simulink model "Tx_Rx"  (R2020a)
settings: Solver=VariableStepAuto  StartTime=0.0  StopTime=640e-9  RelTol=1e-3
libraries: msbUtilities x102, simulink_extras x15, dspswit3 x4, dspsigops x2
(part 1 of 3)
settings Model: Creator=lenovo  LastModifiedBy=dell

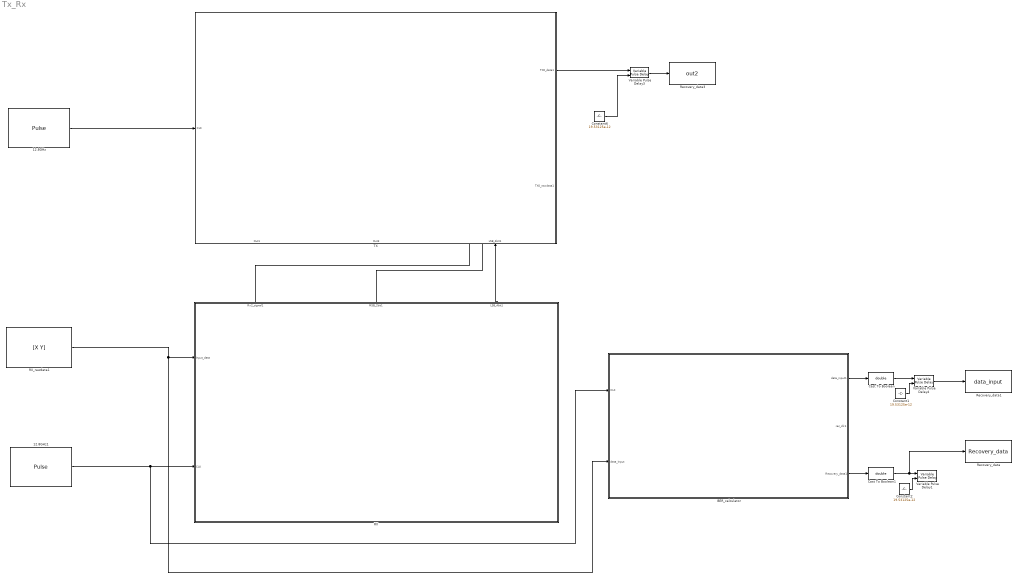
== system Tx_Rx ==
  12.8GHz : DiscretePulseGenerator  PulseType=Time based  Period=78.125e-12  PulseWidth=50
  12.8GHz1 : DiscretePulseGenerator  PulseType=Time based  Period=78.125e-12  PulseWidth=50
  BER_calculator : Subsystem
  Cast To Boolean : DataTypeConversion  OutDataTypeStr=double
  Cast To Boolean1 : DataTypeConversion  OutDataTypeStr=double
  Constant1 : Constant  Value=19.53125e-12
  Constant2 : Constant  Value=19.53125e-12
  Constant6 : Constant  Value=19.53125e-12
  RX : Subsystem
      settings: PortSchema="{\"entries\":[{\"content\":{\"sides\":[{\"content\":{\"connectorIds\":[]},\"type\":\"ConnectorPlacement.EquallySpacedRectSide\",\"uuid\":\"83fb874e-4081-4857-a545-3ede401996a7\"},{\"content\":{\"connectorIds\":[\"Out1\",\"Out2\",\"Out3\"],\"side\":\"RIGHT\"},\"type\":\"ConnectorPlacement.EquallySpacedRectSide\",\"uuid\":\"baf7f71f-d39c-46fb-b6e7-a302eb8d75df\"},{\"content\":{\"connectorIds\":[\"In1\",\"In2\"],\"side\":\"TOP\"},\"type\":\"ConnectorPlacement.EquallySpacedRectSide\",\"uuid\":\"afee1bbb-74d0-41b9-9455-dab1a6c8e3ec\"}]},\"type\":\"ConnectorPlacement.EquallySpacedConnector\",\"uuid\":\"642b16a5-7b6d-4c37-b7c9-a415dc76cc31\"}],\"packageUris\":[\"http://schema.mathworks.com/mf0/Connector/19700101\"],\"version\":\"1.0\"}"
  RX_rawdata1 : FromWorkspace  VariableName=[X Y]  SampleTime=1.220703125e-12  OutputAfterFinalValue=Setting to zero
  Recovery_data : ToWorkspace  VariableName=Recovery_data  SampleTime=39.0625e-12
  Recovery_data1 : ToWorkspace  VariableName=data_input  SampleTime=39.0625e-12
  Recovery_data3 : ToWorkspace  VariableName=out2  SampleTime=1.220703125e-12
  TX : Subsystem
      settings: PortSchema="{\"entries\":[{\"content\":{\"sides\":[{\"content\":{\"connectorIds\":[\"In1\"]},\"type\":\"ConnectorPlacement.EquallySpacedRectSide\",\"uuid\":\"015516c1-0694-4ea3-8d09-2e9ebfdbbb85\"},{\"content\":{\"connectorIds\":[\"Out1\",\"Out2\"],\"side\":\"RIGHT\"},\"type\":\"ConnectorPlacement.EquallySpacedRectSide\",\"uuid\":\"1aa9a16b-7d5d-42f6-9915-24b091a58ba3\"},{\"content\":{\"connectorIds\":[],\"side\":\"TOP\"},\"type\":\"ConnectorPlacement.EquallySpacedRectSide\",\"uuid\":\"832d516b-3e05-4688-bd1f-ad20964f9464\"},{\"content\":{\"connectorIds\":[\"Out3\",\"Out4\",\"In2\"],\"side\":\"BOTTOM\"},\"type\":\"ConnectorPlacement.EquallySpacedRectSide\",\"uuid\":\"9f801a49-c84e-4cc8-8250-723df3cdc162\"}]},\"type\":\"ConnectorPlacement.EquallySpacedConnector\",\"uuid\":\"0b900d77-a4a0-41af-8f34-5efdc4bff0ed\"}],\"packageUris\":[\"http://schema.mathworks.com/mf0/Connector/19700101\"],\"version\":\"1.0\"}"
  Variable Pulse Delay1 : msbUtilities/Variable Pulse Delay  InitialInput=0  BufferSize=100
      settings: SourceProductBaseCode=AM
  Variable Pulse Delay3 : msbUtilities/Variable Pulse Delay  InitialInput=0  BufferSize=100
      settings: SourceProductBaseCode=AM
  Variable Pulse Delay4 : msbUtilities/Variable Pulse Delay  InitialInput=0  BufferSize=100
      settings: SourceProductBaseCode=AM
  wires:
  12.8GHz/1 -> TX/1(CLK)
  RX/2(MSB_2bit1) -> ?
  RX/3(LSB_4bit1) -> TX/2(LSB_4bit1)
  Cast To Boolean/1 -> Variable Pulse Delay4/1
  BER_calculator/1(data_input1) -> Cast To Boolean/1
  BER_calculator/3(Recovery_data1) -> Cast To Boolean1/1
  TX/1(TX0_data1) -> Variable Pulse Delay3/1
  Constant1/1 -> Variable Pulse Delay4/2
  Constant2/1 -> Variable Pulse Delay1/2
  Constant6/1 -> Variable Pulse Delay3/2
  Variable Pulse Delay4/1 -> Recovery_data1/1
  RX_rawdata1/1 -> RX/2(Input_data), BER_calculator/2(data_Input)
  Variable Pulse Delay3/1 -> Recovery_data3/1
  Cast To Boolean1/1 -> Recovery_data/1, Variable Pulse Delay1/1
  RX/1(Rx2_signal1) -> ?
  12.8GHz1/1 -> RX/1(CLK), BER_calculator/1(CLK)

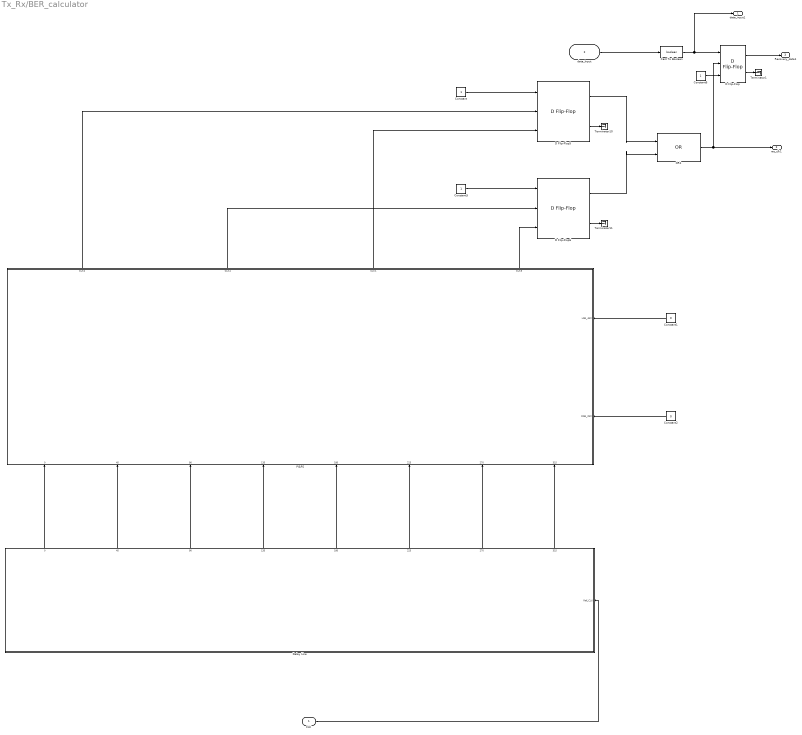
== system Tx_Rx/BER_calculator ==
  CLK : Inport
  data_Input : Inport  Port=2
  Cast To Boolean : DataTypeConversion  OutDataTypeStr=boolean  SaturateOnIntegerOverflow=on
  Constant : Constant  OutDataTypeStr=boolean
  Constant1 : Constant  Value=0
  Constant2 : Constant  Value=0
  Constant5 : Constant  OutDataTypeStr=boolean
  Constant6 : Constant
  D Flip-Flop : simulink_extras/Flip Flops/D Flip-Flop
  D Flip-Flop5 : simulink_extras/Flip Flops/D Flip-Flop
  D Flip-Flop6 : simulink_extras/Flip Flops/D Flip-Flop
  Delay Line : Subsystem
      settings: PortSchema="{\"entries\":[{\"content\":{\"sides\":[{\"content\":{\"connectorIds\":[]},\"type\":\"ConnectorPlacement.EquallySpacedRectSide\",\"uuid\":\"17715945-2f43-441d-a115-2844f3edc5ab\"},{\"content\":{\"connectorIds\":[\"Out1\",\"Out2\",\"Out3\",\"Out4\",\"Out5\",\"Out6\",\"Out7\",\"Out8\"],\"side\":\"RIGHT\"},\"type\":\"ConnectorPlacement.EquallySpacedRectSide\",\"uuid\":\"7a6b272c-522d-4f6f-8262-5d1e4fb1347e\"},{\"content\":{\"connectorIds\":[],\"side\":\"TOP\"},\"type\":\"ConnectorPlacement.EquallySpacedRectSide\",\"uuid\":\"b61d6799-c57d-442f-9306-3db447d9db5e\"},{\"content\":{\"connectorIds\":[\"In1\"],\"side\":\"BOTTOM\"},\"type\":\"ConnectorPlacement.EquallySpacedRectSide\",\"uuid\":\"a0363d09-4ed5-4ac7-969a-2675e4ff1c82\"}]},\"type\":\"ConnectorPlacement.EquallySpacedConnector\",\"uuid\":\"cc79cbb1-d325-49b3-99c0-84c62ae106b4\"}],\"packageUris\":[\"http://schema.mathworks.com/mf0/Connector/19700101\"],\"version\":\"1.0\"}"
  OR1 : Logic  Operator=OR  IconShape=distinctive  AllPortsSameDT=off  OutDataTypeStr=boolean
  PI&PS : Subsystem
      settings: PortSchema="{\"entries\":[{\"content\":{\"sides\":[{\"content\":{\"connectorIds\":[\"In1\",\"In2\",\"In3\",\"In4\",\"In5\",\"In6\",\"In7\",\"In8\"]},\"type\":\"ConnectorPlacement.EquallySpacedRectSide\",\"uuid\":\"c3144821-6f6e-40a9-835d-6ad4fe81ba1a\"},{\"content\":{\"connectorIds\":[\"Out1\",\"Out2\",\"Out3\",\"Out4\"],\"side\":\"RIGHT\"},\"type\":\"ConnectorPlacement.EquallySpacedRectSide\",\"uuid\":\"c5d765ba-0377-4d3a-935f-2ec17305d378\"},{\"content\":{\"connectorIds\":[],\"side\":\"TOP\"},\"type\":\"ConnectorPlacement.EquallySpacedRectSide\",\"uuid\":\"d3f7769c-650b-40bf-9d93-273176cc561b\"},{\"content\":{\"connectorIds\":[\"In9\",\"In10\"],\"side\":\"BOTTOM\"},\"type\":\"ConnectorPlacement.EquallySpacedRectSide\",\"uuid\":\"a470fd3a-9db3-4464-8333-737015181753\"}]},\"type\":\"ConnectorPlacement.EquallySpacedConnector\",\"uuid\":\"35d4e0ec-a507-4c3c-8f19-3aa1177e9fb1\"}],\"packageUris\":[\"http://schema.mathworks.com/mf0/Connector/19700101\"],\"version\":\"1.0\"}"
  Terminator1 : Terminator
  Terminator10 : Terminator
  Terminator11 : Terminator
  data_input1 : Outport
  rec_clk1 : Outport  Port=2
  Recovery_data1 : Outport  Port=3
  wires:
  Constant1/1 -> PI&PS/10(LSB_4bit)
  Delay Line/6(225) -> PI&PS/6(225)
  D Flip-Flop6/1 -> OR1/2
  Delay Line/4(135) -> PI&PS/4(135)
  OR1/1 -> rec_clk1/1, D Flip-Flop/2
  D Flip-Flop/1 -> Recovery_data1/1
  Delay Line/8(315) -> PI&PS/8(315)
  D Flip-Flop5/1 -> OR1/1
  D Flip-Flop/2 -> Terminator1/1
  Constant/1 -> D Flip-Flop5/1
  Delay Line/5(180) -> PI&PS/5(180)
  Delay Line/1(0) -> PI&PS/1(0)
  Delay Line/7(270) -> PI&PS/7(270)
  Delay Line/3(90) -> PI&PS/3(90)
  Delay Line/2(45) -> PI&PS/2(45)
  D Flip-Flop5/2 -> Terminator10/1
  Constant2/1 -> PI&PS/9(MSB_2bit)
  Cast To Boolean/1 -> data_input1/1, D Flip-Flop/1
  Constant6/1 -> D Flip-Flop/3
  Constant5/1 -> D Flip-Flop6/1
  D Flip-Flop6/2 -> Terminator11/1
  CLK/1 -> Delay Line/1(Ref_CLK)
  PI&PS/1(CLK2) -> D Flip-Flop5/2
  PI&PS/2(CLK4) -> D Flip-Flop6/2
  PI&PS/3(CLK1) -> D Flip-Flop5/3
  PI&PS/4(CLK3) -> D Flip-Flop6/3
  data_Input/1 -> Cast To Boolean/1

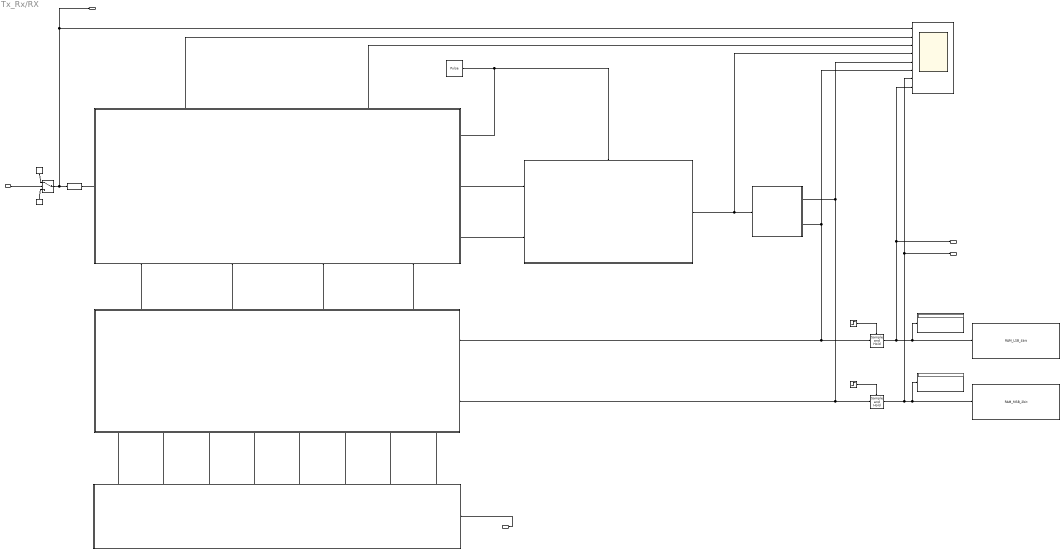
== system Tx_Rx/RX ==
  CLK : Inport
  Input_data : Inport  Port=2
  400MHz_2.5ns(64bit) : DiscretePulseGenerator  PulseType=Time based  Period=2.5e-9  PulseWidth=50
  BBPD : Subsystem
      settings: PortSchema="{\"entries\":[{\"content\":{\"sides\":[{\"content\":{\"connectorIds\":[\"In1\",\"In2\",\"In3\",\"In4\"]},\"type\":\"ConnectorPlacement.EquallySpacedRectSide\",\"uuid\":\"4d1cad8b-8e97-4fbf-a626-ef2f4f4ea09d\"},{\"content\":{\"connectorIds\":[\"Out1\",\"Out2\"],\"side\":\"RIGHT\"},\"type\":\"ConnectorPlacement.EquallySpacedRectSide\",\"uuid\":\"70bd7e42-2a15-424f-9b63-5cb51ecd922a\"},{\"content\":{\"connectorIds\":[\"In5\"],\"side\":\"TOP\"},\"type\":\"ConnectorPlacement.EquallySpacedRectSide\",\"uuid\":\"24ba8e4e-d2ba-4979-9b2f-b5eeebb57a1c\"},{\"content\":{\"connectorIds\":[\"Out3\",\"Out4\",\"In6\"],\"side\":\"BOTTOM\"},\"type\":\"ConnectorPlacement.EquallySpacedRectSide\",\"uuid\":\"fcecb8f5-383e-4216-80da-14864d9f0171\"}]},\"type\":\"ConnectorPlacement.EquallySpacedConnector\",\"uuid\":\"bced9882-2d17-491b-9f35-fead766c42db\"}],\"packageUris\":[\"http://schema.mathworks.com/mf0/Connector/19700101\"],\"version\":\"1.0\"}"
  Binary_divider : MATLAB Function  TreatAsAtomicUnit=on
  Cast To Boolean : DataTypeConversion  OutDataTypeStr=boolean  SaturateOnIntegerOverflow=on
  Constant3 : Constant
  Constant4 : Constant  Value=0
  Data Store Write : DataStoreWrite  DataStoreName=RAM_LSB_4bit
  Data Store Write1 : DataStoreWrite  DataStoreName=RAM_MSB_2bit
  Delay Line : Subsystem
      settings: PortSchema="{\"entries\":[{\"content\":{\"sides\":[{\"content\":{\"connectorIds\":[]},\"type\":\"ConnectorPlacement.EquallySpacedRectSide\",\"uuid\":\"17715945-2f43-441d-a115-2844f3edc5ab\"},{\"content\":{\"connectorIds\":[\"Out1\",\"Out2\",\"Out3\",\"Out4\",\"Out5\",\"Out6\",\"Out7\",\"Out8\"],\"side\":\"RIGHT\"},\"type\":\"ConnectorPlacement.EquallySpacedRectSide\",\"uuid\":\"7a6b272c-522d-4f6f-8262-5d1e4fb1347e\"},{\"content\":{\"connectorIds\":[],\"side\":\"TOP\"},\"type\":\"ConnectorPlacement.EquallySpacedRectSide\",\"uuid\":\"b61d6799-c57d-442f-9306-3db447d9db5e\"},{\"content\":{\"connectorIds\":[\"In1\"],\"side\":\"BOTTOM\"},\"type\":\"ConnectorPlacement.EquallySpacedRectSide\",\"uuid\":\"a0363d09-4ed5-4ac7-969a-2675e4ff1c82\"}]},\"type\":\"ConnectorPlacement.EquallySpacedConnector\",\"uuid\":\"cc79cbb1-d325-49b3-99c0-84c62ae106b4\"}],\"packageUris\":[\"http://schema.mathworks.com/mf0/Connector/19700101\"],\"version\":\"1.0\"}"
  Display2 : Display
  Display3 : Display
  FSM : Stateflow chart  TreatAsAtomicUnit=on
  PI&PS : Subsystem
      settings: PortSchema="{\"entries\":[{\"content\":{\"sides\":[{\"content\":{\"connectorIds\":[\"In1\",\"In2\",\"In3\",\"In4\",\"In5\",\"In6\",\"In7\",\"In8\"]},\"type\":\"ConnectorPlacement.EquallySpacedRectSide\",\"uuid\":\"c3144821-6f6e-40a9-835d-6ad4fe81ba1a\"},{\"content\":{\"connectorIds\":[\"Out1\",\"Out2\",\"Out3\",\"Out4\"],\"side\":\"RIGHT\"},\"type\":\"ConnectorPlacement.EquallySpacedRectSide\",\"uuid\":\"c5d765ba-0377-4d3a-935f-2ec17305d378\"},{\"content\":{\"connectorIds\":[],\"side\":\"TOP\"},\"type\":\"ConnectorPlacement.EquallySpacedRectSide\",\"uuid\":\"d3f7769c-650b-40bf-9d93-273176cc561b\"},{\"content\":{\"connectorIds\":[\"In9\",\"In10\"],\"side\":\"BOTTOM\"},\"type\":\"ConnectorPlacement.EquallySpacedRectSide\",\"uuid\":\"a470fd3a-9db3-4464-8333-737015181753\"}]},\"type\":\"ConnectorPlacement.EquallySpacedConnector\",\"uuid\":\"35d4e0ec-a507-4c3c-8f19-3aa1177e9fb1\"}],\"packageUris\":[\"http://schema.mathworks.com/mf0/Connector/19700101\"],\"version\":\"1.0\"}"
  Sample and Hold : dspsigops/Sample and Hold  trig=Rising edge  initCond=0  latchinput=off
  Sample and Hold1 : dspsigops/Sample and Hold  trig=Rising edge  initCond=0  latchinput=off
  Scope : Scope  NumInputPorts=8
  Step : Step  Time=128e-9
  Step1 : Step  Time=128e-9
  Switch : Switch  Criteria=u2 > Threshold  Threshold=0.5
  Rx2_signal1 : Outport
  MSB_2bit1 : Outport  Port=2
  LSB_4bit1 : Outport  Port=3
  wires:
  Cast To Boolean/1 -> BBPD/5(DATA_in)
  Binary_divider/1(MSB_2bit) -> Scope/5, Sample and Hold1/1, PI&PS/9(MSB_2bit)
  Switch/1 -> Rx2_signal1/1, Scope/1, Cast To Boolean/1
  PI&PS/3(CLK3) -> BBPD/3(CLK3)
  BBPD/4(E) -> FSM/1(E)
  Delay Line/2(45) -> PI&PS/2(45)
  BBPD/3(S) -> FSM/2(S)
  PI&PS/4(CLK4) -> BBPD/4(CLK4)
  Delay Line/6(225) -> PI&PS/6(225)
  Sample and Hold1/1 -> MSB_2bit1/1, Scope/7, Display3/1, Data Store Write1/1
  BBPD/2(DOWN_64bit) -> Scope/3
  Constant4/1 -> Switch/3
  Delay Line/8(315) -> PI&PS/8(315)
  BBPD/1(UP_64bit) -> Scope/2
  Delay Line/4(135) -> PI&PS/4(135)
  Delay Line/5(180) -> PI&PS/5(180)
  Delay Line/3(90) -> PI&PS/3(90)
  400MHz_2.5ns(64bit)/1 -> FSM/Trigger, BBPD/6(CLK_2.5ns)
  Delay Line/1(0) -> PI&PS/1(0)
  Step/1 -> Sample and Hold/Trigger
  PI&PS/2(CLK2) -> BBPD/2(CLK2)
  FSM/1(DATA) -> Scope/4, Binary_divider/1(DATA)
  Binary_divider/2(LSB_4bit) -> Scope/6, Sample and Hold/1, PI&PS/10(LSB_4bit)
  Delay Line/7(270) -> PI&PS/7(270)
  Sample and Hold/1 -> LSB_4bit1/1, Scope/8, Display2/1, Data Store Write/1
  Constant3/1 -> Switch/1
  Step1/1 -> Sample and Hold1/Trigger
  PI&PS/1(CLK1) -> BBPD/1(CLK1)
  Input_data/1 -> Switch/2
  CLK/1 -> Delay Line/1(Ref_CLK)

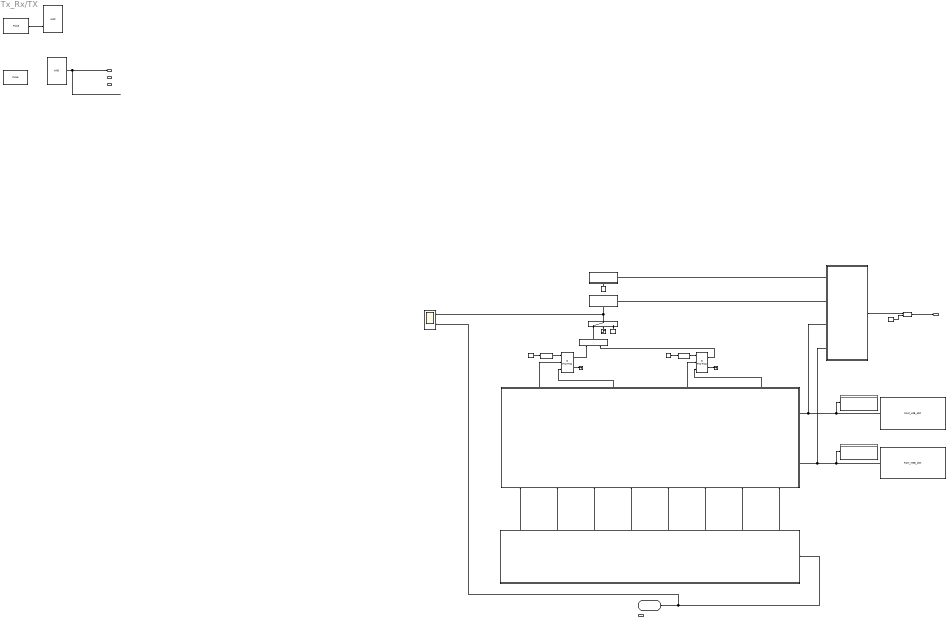
== system Tx_Rx/TX ==
  CLK : Inport
  LSB_4bit1 : Inport  Port=2
  " De Bruijn序列生成器" : Subsystem
  AND : Logic  IconShape=distinctive  AllPortsSameDT=off  OutDataTypeStr=boolean
  AND1 : Logic  IconShape=distinctive  AllPortsSameDT=off  OutDataTypeStr=boolean
  Cast To Boolean : DataTypeConversion  OutDataTypeStr=boolean
  Cast To Boolean1 : DataTypeConversion  OutDataTypeStr=boolean
  Constant1 : Constant
  Constant2 : Constant
  Constant3 : Constant
  Constant6 : Constant  Value=39.0625e-12
  D Flip-Flop15 : simulink_extras/Flip Flops/D Flip-Flop
  D Flip-Flop16 : simulink_extras/Flip Flops/D Flip-Flop
  Data Store Read : DataStoreRead  DataStoreName=RAM_LSB_4bit
  Data Store Read1 : DataStoreRead  DataStoreName=RAM_MSB_2bit
  De Bruijn序列生成器 : Subsystem
  Delay Line1 : Subsystem
      settings: PortSchema="{\"entries\":[{\"content\":{\"sides\":[{\"content\":{\"connectorIds\":[]},\"type\":\"ConnectorPlacement.EquallySpacedRectSide\",\"uuid\":\"17715945-2f43-441d-a115-2844f3edc5ab\"},{\"content\":{\"connectorIds\":[\"Out1\",\"Out2\",\"Out3\",\"Out4\",\"Out5\",\"Out6\",\"Out7\",\"Out8\"],\"side\":\"RIGHT\"},\"type\":\"ConnectorPlacement.EquallySpacedRectSide\",\"uuid\":\"7a6b272c-522d-4f6f-8262-5d1e4fb1347e\"},{\"content\":{\"connectorIds\":[],\"side\":\"TOP\"},\"type\":\"ConnectorPlacement.EquallySpacedRectSide\",\"uuid\":\"b61d6799-c57d-442f-9306-3db447d9db5e\"},{\"content\":{\"connectorIds\":[\"In1\"],\"side\":\"BOTTOM\"},\"type\":\"ConnectorPlacement.EquallySpacedRectSide\",\"uuid\":\"a0363d09-4ed5-4ac7-969a-2675e4ff1c82\"}]},\"type\":\"ConnectorPlacement.EquallySpacedConnector\",\"uuid\":\"cc79cbb1-d325-49b3-99c0-84c62ae106b4\"}],\"packageUris\":[\"http://schema.mathworks.com/mf0/Connector/19700101\"],\"version\":\"1.0\"}"
  Display : Display
  Display1 : Display
  MATLAB Function : MATLAB Function  TreatAsAtomicUnit=on
  OR2 : Logic  Operator=OR  IconShape=distinctive  AllPortsSameDT=off  OutDataTypeStr=boolean
  PI&PS1 : Subsystem
      settings: PortSchema="{\"entries\":[{\"content\":{\"sides\":[{\"content\":{\"connectorIds\":[\"In1\",\"In2\",\"In3\",\"In4\",\"In5\",\"In6\",\"In7\",\"In8\"]},\"type\":\"ConnectorPlacement.EquallySpacedRectSide\",\"uuid\":\"c3144821-6f6e-40a9-835d-6ad4fe81ba1a\"},{\"content\":{\"connectorIds\":[\"Out1\",\"Out2\",\"Out3\",\"Out4\"],\"side\":\"RIGHT\"},\"type\":\"ConnectorPlacement.EquallySpacedRectSide\",\"uuid\":\"c5d765ba-0377-4d3a-935f-2ec17305d378\"},{\"content\":{\"connectorIds\":[],\"side\":\"TOP\"},\"type\":\"ConnectorPlacement.EquallySpacedRectSide\",\"uuid\":\"d3f7769c-650b-40bf-9d93-273176cc561b\"},{\"content\":{\"connectorIds\":[\"In9\",\"In10\"],\"side\":\"BOTTOM\"},\"type\":\"ConnectorPlacement.EquallySpacedRectSide\",\"uuid\":\"a470fd3a-9db3-4464-8333-737015181753\"}]},\"type\":\"ConnectorPlacement.EquallySpacedConnector\",\"uuid\":\"35d4e0ec-a507-4c3c-8f19-3aa1177e9fb1\"}],\"packageUris\":[\"http://schema.mathworks.com/mf0/Connector/19700101\"],\"version\":\"1.0\"}"
  Peroid_65ns : DiscretePulseGenerator  PulseType=Time based  Period=130e-9  PulseWidth=600/13
  Peroid_65ns1 : DiscretePulseGenerator  PulseType=Time based  Period=130e-9  PulseWidth=600/13
  Pulse Generator : DiscretePulseGenerator  PulseType=Time based  Period=39.0625e-12  PulseWidth=50  PhaseDelay=1e-100
  Scope : Scope  NumInputPorts=2
  Step : Step  Time=129960.9375e-12
  Switch : Switch  Criteria=u2 > Threshold
  Terminator : Terminator
  Terminator1 : Terminator
  Variable Pulse Delay3 : msbUtilities/Variable Pulse Delay  InitialInput=0  BufferSize=100
      settings: SourceProductBaseCode=AM
  TX0_data1 : Outport
  TX0_rawdata1 : Outport  Port=2
  Out1 : Outport  Port=3
  Out3 : Outport  Port=4
  wires:
  Pulse Generator/1 -> De Bruijn序列生成器/Trigger
  Constant1/1 -> Cast To Boolean/1
  Delay Line1/8(315) -> PI&PS1/8(315)
  Delay Line1/6(225) -> PI&PS1/6(225)
  Delay Line1/3(90) -> PI&PS1/3(90)
  PI&PS1/3(CLK3) -> D Flip-Flop16/2
  D Flip-Flop16/2 -> Terminator1/1
  Delay Line1/1(0) -> PI&PS1/1(0)
  Delay Line1/7(270) -> PI&PS1/7(270)
  PI&PS1/1(CLK1) -> D Flip-Flop15/2
  AND1/1 -> TX0_rawdata1/1
  D Flip-Flop16/1 -> OR2/2
  Delay Line1/2(45) -> PI&PS1/2(45)
  Delay Line1/4(135) -> PI&PS1/4(135)
  PI&PS1/4(CLK2) -> D Flip-Flop16/3
  Delay Line1/5(180) -> PI&PS1/5(180)
  Constant2/1 -> Cast To Boolean1/1
  OR2/1 -> Switch/1
  D Flip-Flop15/2 -> Terminator/1
  D Flip-Flop15/1 -> OR2/1
  Data Store Read/1 -> Display/1, PI&PS1/10(LSB_4bit), MATLAB Function/3(LSB_4bit)
  PI&PS1/2(CLK4) -> D Flip-Flop15/3
  Constant3/1 -> Switch/3
  Switch/1 -> " De Bruijn序列生成器"/Trigger, Scope/1
  Cast To Boolean1/1 -> D Flip-Flop16/1
  Data Store Read1/1 -> PI&PS1/9(MSB_2bit), MATLAB Function/4(MSB_2bit), Display1/1
  Cast To Boolean/1 -> D Flip-Flop15/1
  Step/1 -> Switch/2
  CLK/1 -> Scope/2, Delay Line1/1(Ref_CLK)
  Peroid_65ns/1 -> AND/2
  De Bruijn序列生成器/1(DB_seq) -> MATLAB Function/1(data_in_ref)
  " De Bruijn序列生成器"/1(DB_seq) -> MATLAB Function/2(data_in_change)
  Constant6/1 -> Variable Pulse Delay3/2
  MATLAB Function/1(data_out) -> Variable Pulse Delay3/1
  Variable Pulse Delay3/1 -> TX0_data1/1

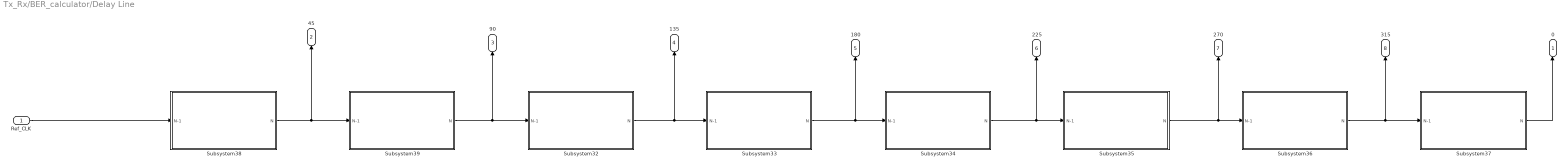
== system Tx_Rx/BER_calculator/Delay Line ==
  Ref_CLK : Inport
  Subsystem32 : Subsystem
  Subsystem33 : Subsystem
  Subsystem34 : Subsystem
  Subsystem35 : Subsystem
  Subsystem36 : Subsystem
  Subsystem37 : Subsystem
  Subsystem38 : Subsystem
  Subsystem39 : Subsystem
  0 : Outport
  45 : Outport  Port=2
  90 : Outport  Port=3
  135 : Outport  Port=4
  180 : Outport  Port=5
  225 : Outport  Port=6
  270 : Outport  Port=7
  315 : Outport  Port=8
  wires:
  Subsystem38/1(N) -> Subsystem39/1(N-1), 45/1
  Subsystem32/1(N) -> 135/1, Subsystem33/1(N-1)
  Subsystem33/1(N) -> 180/1, Subsystem34/1(N-1)
  Subsystem39/1(N) -> Subsystem32/1(N-1), 90/1
  Subsystem34/1(N) -> Subsystem35/1(N-1), 225/1
  Subsystem36/1(N) -> Subsystem37/1(N-1), 315/1
  Subsystem35/1(N) -> Subsystem36/1(N-1), 270/1
  Ref_CLK/1 -> Subsystem38/1(N-1)
  Subsystem37/1(N) -> 0/1

== system Tx_Rx/BER_calculator/PI&PS ==
  0 : Inport
  45 : Inport  Port=2
  90 : Inport  Port=3
  135 : Inport  Port=4
  180 : Inport  Port=5
  225 : Inport  Port=6
  270 : Inport  Port=7
  315 : Inport  Port=8
  MSB_2bit : Inport  Port=9
  LSB_4bit : Inport  Port=10
  Phase Interpolator : Subsystem
      settings: PortSchema="{\"entries\":[{\"content\":{\"sides\":[{\"content\":{\"connectorIds\":[\"In1\",\"In2\"]},\"type\":\"ConnectorPlacement.EquallySpacedRectSide\",\"uuid\":\"dfcd2233-b4c1-4cf7-8cd6-e1b13d3e96a6\"},{\"content\":{\"connectorIds\":[\"Out1\",\"Out2\",\"Out3\",\"Out4\"],\"side\":\"RIGHT\"},\"type\":\"ConnectorPlacement.EquallySpacedRectSide\",\"uuid\":\"fcdf078d-3861-4110-b2e2-4d0c398726ab\"},{\"content\":{\"connectorIds\":[],\"side\":\"TOP\"},\"type\":\"ConnectorPlacement.EquallySpacedRectSide\",\"uuid\":\"b2ad88e9-f4d9-48df-8a2b-60ffe78c0d74\"},{\"content\":{\"connectorIds\":[\"In3\"],\"side\":\"BOTTOM\"},\"type\":\"ConnectorPlacement.EquallySpacedRectSide\",\"uuid\":\"39ef07a5-295e-41ed-8fed-e3929d4bc7fe\"}]},\"type\":\"ConnectorPlacement.EquallySpacedConnector\",\"uuid\":\"6304a2bd-355b-45e4-9c14-1a54db954efb\"}],\"packageUris\":[\"http://schema.mathworks.com/mf0/Connector/19700101\"],\"version\":\"1.0\"}"
  Phase Selector : Subsystem
      settings: PortSchema="{\"entries\":[{\"content\":{\"sides\":[{\"content\":{\"connectorIds\":[\"In1\",\"In2\",\"In3\",\"In4\",\"In5\",\"In6\",\"In7\",\"In8\"]},\"type\":\"ConnectorPlacement.EquallySpacedRectSide\",\"uuid\":\"7503323e-6ee4-44ff-b04d-f2dbeaa5c6ec\"},{\"content\":{\"connectorIds\":[\"Out1\",\"Out2\"],\"side\":\"RIGHT\"},\"type\":\"ConnectorPlacement.EquallySpacedRectSide\",\"uuid\":\"41a61174-d293-4df5-a84f-f0e93c8bdc8e\"},{\"content\":{\"connectorIds\":[],\"side\":\"TOP\"},\"type\":\"ConnectorPlacement.EquallySpacedRectSide\",\"uuid\":\"fa0b14f5-0011-4a0b-b494-1db998357d4b\"},{\"content\":{\"connectorIds\":[\"In9\"],\"side\":\"BOTTOM\"},\"type\":\"ConnectorPlacement.EquallySpacedRectSide\",\"uuid\":\"f33c2322-8ee6-4a57-a447-492661ada981\"}]},\"type\":\"ConnectorPlacement.EquallySpacedConnector\",\"uuid\":\"0b93855a-73ca-4614-8a61-5e157f0666c2\"}],\"packageUris\":[\"http://schema.mathworks.com/mf0/Connector/19700101\"],\"version\":\"1.0\"}"
  CLK2 : Outport
  CLK4 : Outport  Port=2
  CLK1 : Outport  Port=3
  CLK3 : Outport  Port=4
  wires:
  0/1 -> Phase Selector/1(0)
  225/1 -> Phase Selector/6(225)
  Phase Selector/2(CLK_s3) -> Phase Interpolator/2(CLK_s3)
  Phase Selector/1(CLK_s1) -> Phase Interpolator/1(CLK_s1)
  315/1 -> Phase Selector/8(315)
  45/1 -> Phase Selector/2(45)
  270/1 -> Phase Selector/7(270)
  135/1 -> Phase Selector/4(135)
  90/1 -> Phase Selector/3(90)
  LSB_4bit/1 -> Phase Interpolator/3(LSB_4bit)
  MSB_2bit/1 -> Phase Selector/9(MSB_2bit)
  Phase Interpolator/2(CLK4) -> CLK4/1
  Phase Interpolator/1(CLK2) -> CLK2/1
  180/1 -> Phase Selector/5(180)
  Phase Interpolator/3(CLK1) -> CLK1/1
  Phase Interpolator/4(CLK3) -> CLK3/1

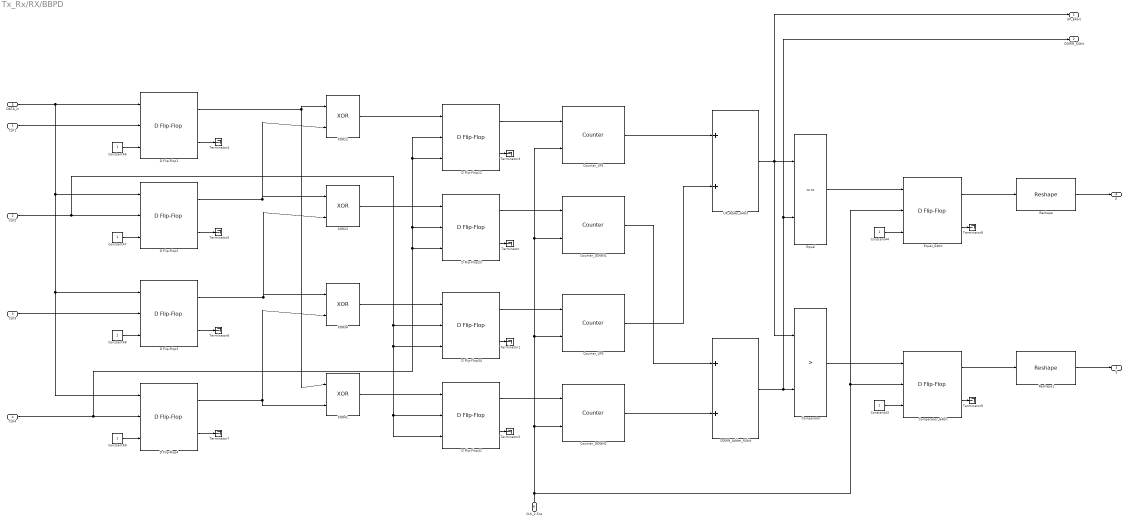
== system Tx_Rx/RX/BBPD ==
  CLK1 : Inport
  CLK2 : Inport  Port=2
  CLK3 : Inport  Port=3
  CLK4 : Inport  Port=4
  DATA_in : Inport  Port=5
  CLK_2.5ns : Inport  Port=6
  Comparator : RelationalOperator  Operator=>  OutDataTypeStr=boolean  RndMeth=Simplest
  Comparator_64bit : simulink_extras/Flip Flops/D Flip-Flop
  Constant{43..44,46..49} (6 alike) : Constant
  Counter_DOWN1 : dspswit3/Counter  Direction=Up  CountEvent=Rising edge  CounterSize=User defined  MaxCount=255  InitialCount=0  Output=Count  HitValue=32  ResetInput=on  SamplesPerFrame=1  Ts=1  CntDtype=double  HitDtype=Logical
  Counter_DOWN2 : dspswit3/Counter  Direction=Up  CountEvent=Rising edge  CounterSize=User defined  MaxCount=255  InitialCount=0  Output=Count  HitValue=32  ResetInput=on  SamplesPerFrame=1  Ts=1  CntDtype=double  HitDtype=Logical
  Counter_UP1 : dspswit3/Counter  Direction=Up  CountEvent=Rising edge  CounterSize=User defined  MaxCount=255  InitialCount=0  Output=Count  HitValue=32  ResetInput=on  SamplesPerFrame=1  Ts=1  CntDtype=double  HitDtype=Logical
  Counter_UP2 : dspswit3/Counter  Direction=Up  CountEvent=Rising edge  CounterSize=User defined  MaxCount=255  InitialCount=0  Output=Count  HitValue=32  ResetInput=on  SamplesPerFrame=1  Ts=1  CntDtype=double  HitDtype=Logical
  D Flip-Flop{1..4,12,23,34,41} (8 alike) : simulink_extras/Flip Flops/D Flip-Flop
  DOWN_Adder_64bit : Sum
  Equal : RelationalOperator  Operator===  OutDataTypeStr=boolean  RndMeth=Simplest
  Equal_64bit : simulink_extras/Flip Flops/D Flip-Flop
  Reshape : Reshape  OutputDimensions=1
  Reshape1 : Reshape  OutputDimensions=1
  Terminator{,1..9} (10 alike) : Terminator
  UP_Adder_64bit : Sum
  XOR{12,23,34,41} (4 alike) : Logic  Operator=XOR  IconShape=distinctive  AllPortsSameDT=off  OutDataTypeStr=boolean
  UP_64bit : Outport
  DOWN_64bit : Outport  Port=2
  S : Outport  Port=3
  E : Outport  Port=4
  wires:
  Equal_64bit/1 -> Reshape/1
  Constant46/1 -> D Flip-Flop1/3
  Comparator_64bit/2 -> Terminator9/1
  CLK1/1 -> D Flip-Flop1/2
  DATA_in/1 -> D Flip-Flop4/1, D Flip-Flop3/1, D Flip-Flop2/1, D Flip-Flop1/1
  Counter_DOWN2/1 -> DOWN_Adder_64bit/2
  Constant48/1 -> D Flip-Flop3/3
  D Flip-Flop23/2 -> Terminator/1
  Constant47/1 -> D Flip-Flop2/3
  Constant44/1 -> Equal_64bit/3
  D Flip-Flop2/1 -> XOR12/2, XOR23/1
  D Flip-Flop4/1 -> XOR41/2, XOR34/2
  CLK2/1 -> D Flip-Flop2/2, D Flip-Flop34/2, D Flip-Flop41/3, D Flip-Flop41/2, D Flip-Flop34/3
  D Flip-Flop3/1 -> XOR23/2, XOR34/1
  CLK3/1 -> D Flip-Flop3/2
  D Flip-Flop1/1 -> XOR41/1, XOR12/1
  Comparator_64bit/1 -> Reshape1/1
  Constant49/1 -> D Flip-Flop4/3
  D Flip-Flop12/1 -> Counter_UP1/1
  D Flip-Flop12/2 -> Terminator3/1
  CLK_2.5ns/1 -> Comparator_64bit/2, Equal_64bit/2, Counter_DOWN2/2, Counter_UP2/2, Counter_DOWN1/2, Counter_UP1/2
  D Flip-Flop41/2 -> Terminator2/1
  Comparator/1 -> Comparator_64bit/1
  D Flip-Flop41/1 -> Counter_DOWN2/1
  XOR12/1 -> D Flip-Flop12/1
  CLK4/1 -> D Flip-Flop4/2, D Flip-Flop23/3, D Flip-Flop23/2, D Flip-Flop12/2, D Flip-Flop12/3
  XOR41/1 -> D Flip-Flop41/1
  D Flip-Flop34/1 -> Counter_UP2/1
  Constant43/1 -> Comparator_64bit/3
  Counter_DOWN1/1 -> DOWN_Adder_64bit/1
  Counter_UP1/1 -> UP_Adder_64bit/1
  UP_Adder_64bit/1 -> UP_64bit/1, Equal/1, Comparator/1
  Counter_UP2/1 -> UP_Adder_64bit/2
  D Flip-Flop4/2 -> Terminator7/1
  Equal/1 -> Equal_64bit/1
  DOWN_Adder_64bit/1 -> DOWN_64bit/1, Equal/2, Comparator/2
  D Flip-Flop23/1 -> Counter_DOWN1/1
  Equal_64bit/2 -> Terminator8/1
  XOR23/1 -> D Flip-Flop23/1
  XOR34/1 -> D Flip-Flop34/1
  Reshape1/1 -> S/1
  Reshape/1 -> E/1
  D Flip-Flop1/2 -> Terminator4/1
  D Flip-Flop34/2 -> Terminator1/1
  D Flip-Flop3/2 -> Terminator6/1
  D Flip-Flop2/2 -> Terminator5/1

== system Tx_Rx/RX/Delay Line ==
  Ref_CLK : Inport
  Subsystem32 : Subsystem
  Subsystem33 : Subsystem
  Subsystem34 : Subsystem
  Subsystem35 : Subsystem
  Subsystem36 : Subsystem
  Subsystem37 : Subsystem
  Subsystem38 : Subsystem
  Subsystem39 : Subsystem
  0 : Outport
  45 : Outport  Port=2
  90 : Outport  Port=3
  135 : Outport  Port=4
  180 : Outport  Port=5
  225 : Outport  Port=6
  270 : Outport  Port=7
  315 : Outport  Port=8
  wires:
  Subsystem38/1(N) -> Subsystem39/1(N-1), 45/1
  Subsystem32/1(N) -> 135/1, Subsystem33/1(N-1)
  Subsystem33/1(N) -> 180/1, Subsystem34/1(N-1)
  Subsystem39/1(N) -> Subsystem32/1(N-1), 90/1
  Subsystem34/1(N) -> Subsystem35/1(N-1), 225/1
  Subsystem36/1(N) -> Subsystem37/1(N-1), 315/1
  Subsystem35/1(N) -> Subsystem36/1(N-1), 270/1
  Ref_CLK/1 -> Subsystem38/1(N-1)
  Subsystem37/1(N) -> 0/1

== system Tx_Rx/RX/PI&PS ==
  0 : Inport
  45 : Inport  Port=2
  90 : Inport  Port=3
  135 : Inport  Port=4
  180 : Inport  Port=5
  225 : Inport  Port=6
  270 : Inport  Port=7
  315 : Inport  Port=8
  MSB_2bit : Inport  Port=9
  LSB_4bit : Inport  Port=10
  Phase Interpolator : Subsystem
      settings: PortSchema="{\"entries\":[{\"content\":{\"sides\":[{\"content\":{\"connectorIds\":[\"In1\",\"In2\"]},\"type\":\"ConnectorPlacement.EquallySpacedRectSide\",\"uuid\":\"dfcd2233-b4c1-4cf7-8cd6-e1b13d3e96a6\"},{\"content\":{\"connectorIds\":[\"Out1\",\"Out2\",\"Out3\",\"Out4\"],\"side\":\"RIGHT\"},\"type\":\"ConnectorPlacement.EquallySpacedRectSide\",\"uuid\":\"fcdf078d-3861-4110-b2e2-4d0c398726ab\"},{\"content\":{\"connectorIds\":[],\"side\":\"TOP\"},\"type\":\"ConnectorPlacement.EquallySpacedRectSide\",\"uuid\":\"b2ad88e9-f4d9-48df-8a2b-60ffe78c0d74\"},{\"content\":{\"connectorIds\":[\"In3\"],\"side\":\"BOTTOM\"},\"type\":\"ConnectorPlacement.EquallySpacedRectSide\",\"uuid\":\"39ef07a5-295e-41ed-8fed-e3929d4bc7fe\"}]},\"type\":\"ConnectorPlacement.EquallySpacedConnector\",\"uuid\":\"6304a2bd-355b-45e4-9c14-1a54db954efb\"}],\"packageUris\":[\"http://schema.mathworks.com/mf0/Connector/19700101\"],\"version\":\"1.0\"}"
  Phase Selector : Subsystem
      settings: PortSchema="{\"entries\":[{\"content\":{\"sides\":[{\"content\":{\"connectorIds\":[\"In1\",\"In2\",\"In3\",\"In4\",\"In5\",\"In6\",\"In7\",\"In8\"]},\"type\":\"ConnectorPlacement.EquallySpacedRectSide\",\"uuid\":\"7503323e-6ee4-44ff-b04d-f2dbeaa5c6ec\"},{\"content\":{\"connectorIds\":[\"Out1\",\"Out2\"],\"side\":\"RIGHT\"},\"type\":\"ConnectorPlacement.EquallySpacedRectSide\",\"uuid\":\"41a61174-d293-4df5-a84f-f0e93c8bdc8e\"},{\"content\":{\"connectorIds\":[],\"side\":\"TOP\"},\"type\":\"ConnectorPlacement.EquallySpacedRectSide\",\"uuid\":\"fa0b14f5-0011-4a0b-b494-1db998357d4b\"},{\"content\":{\"connectorIds\":[\"In9\"],\"side\":\"BOTTOM\"},\"type\":\"ConnectorPlacement.EquallySpacedRectSide\",\"uuid\":\"f33c2322-8ee6-4a57-a447-492661ada981\"}]},\"type\":\"ConnectorPlacement.EquallySpacedConnector\",\"uuid\":\"0b93855a-73ca-4614-8a61-5e157f0666c2\"}],\"packageUris\":[\"http://schema.mathworks.com/mf0/Connector/19700101\"],\"version\":\"1.0\"}"
  CLK1 : Outport
  CLK2 : Outport  Port=2
  CLK3 : Outport  Port=3
  CLK4 : Outport  Port=4
  wires:
  0/1 -> Phase Selector/1(0)
  225/1 -> Phase Selector/6(225)
  Phase Selector/2(CLK_s3) -> Phase Interpolator/2(CLK_s3)
  Phase Selector/1(CLK_s1) -> Phase Interpolator/1(CLK_s1)
  315/1 -> Phase Selector/8(315)
  45/1 -> Phase Selector/2(45)
  270/1 -> Phase Selector/7(270)
  135/1 -> Phase Selector/4(135)
  90/1 -> Phase Selector/3(90)
  LSB_4bit/1 -> Phase Interpolator/3(LSB_4bit)
  Phase Interpolator/1(CLK1) -> CLK1/1
  MSB_2bit/1 -> Phase Selector/9(MSB_2bit)
  Phase Interpolator/4(CLK4) -> CLK4/1
  Phase Interpolator/3(CLK3) -> CLK3/1
  Phase Interpolator/2(CLK2) -> CLK2/1
  180/1 -> Phase Selector/5(180)

== system Tx_Rx/TX/ De Bruijn序列生成器 ==
  Trigger : TriggerPort  VariantControl=Variant  PortDimensions=1
  MATLAB Function : MATLAB Function  TreatAsAtomicUnit=on
  Memory : Memory  InitialCondition=[1 0 1 0 0 1 1 0 1 1 1 1 0 0 0 0]  InheritSampleTime=on
  DB_seq : Outport
  wires:
  MATLAB Function/1(DB_seq_s) -> DB_seq/1
  MATLAB Function/2(DB_seq_p) -> Memory/1
  Memory/1 -> MATLAB Function/1("DB_seq_p ")

== system Tx_Rx/TX/De Bruijn序列生成器 ==
  Trigger : TriggerPort  VariantControl=Variant  PortDimensions=1
  MATLAB Function : MATLAB Function  TreatAsAtomicUnit=on
  Memory : Memory  InitialCondition=[1 0 1 0 0 1 1 0 1 1 1 1 0 0 0 0]  InheritSampleTime=on
  DB_seq : Outport
  wires:
  MATLAB Function/1(DB_seq_s) -> DB_seq/1
  MATLAB Function/2(DB_seq_p) -> Memory/1
  Memory/1 -> MATLAB Function/1("DB_seq_p ")

== system Tx_Rx/TX/Delay Line1 ==
  Ref_CLK : Inport
  Subsystem32 : Subsystem
  Subsystem33 : Subsystem
  Subsystem34 : Subsystem
  Subsystem35 : Subsystem
  Subsystem36 : Subsystem
  Subsystem37 : Subsystem
  Subsystem38 : Subsystem
  Subsystem39 : Subsystem
  0 : Outport
  45 : Outport  Port=2
  90 : Outport  Port=3
  135 : Outport  Port=4
  180 : Outport  Port=5
  225 : Outport  Port=6
  270 : Outport  Port=7
  315 : Outport  Port=8
  wires:
  Subsystem38/1(N) -> Subsystem39/1(N-1), 45/1
  Subsystem32/1(N) -> 135/1, Subsystem33/1(N-1)
  Subsystem33/1(N) -> 180/1, Subsystem34/1(N-1)
  Subsystem39/1(N) -> Subsystem32/1(N-1), 90/1
  Subsystem34/1(N) -> Subsystem35/1(N-1), 225/1
  Subsystem36/1(N) -> Subsystem37/1(N-1), 315/1
  Subsystem35/1(N) -> Subsystem36/1(N-1), 270/1
  Ref_CLK/1 -> Subsystem38/1(N-1)
  Subsystem37/1(N) -> 0/1

== system Tx_Rx/TX/PI&PS1 ==
  0 : Inport
  45 : Inport  Port=2
  90 : Inport  Port=3
  135 : Inport  Port=4
  180 : Inport  Port=5
  225 : Inport  Port=6
  270 : Inport  Port=7
  315 : Inport  Port=8
  MSB_2bit : Inport  Port=9
  LSB_4bit : Inport  Port=10
  Phase Interpolator : Subsystem
      settings: PortSchema="{\"entries\":[{\"content\":{\"sides\":[{\"content\":{\"connectorIds\":[\"In1\",\"In2\"]},\"type\":\"ConnectorPlacement.EquallySpacedRectSide\",\"uuid\":\"dfcd2233-b4c1-4cf7-8cd6-e1b13d3e96a6\"},{\"content\":{\"connectorIds\":[\"Out1\",\"Out2\",\"Out3\",\"Out4\"],\"side\":\"RIGHT\"},\"type\":\"ConnectorPlacement.EquallySpacedRectSide\",\"uuid\":\"fcdf078d-3861-4110-b2e2-4d0c398726ab\"},{\"content\":{\"connectorIds\":[],\"side\":\"TOP\"},\"type\":\"ConnectorPlacement.EquallySpacedRectSide\",\"uuid\":\"b2ad88e9-f4d9-48df-8a2b-60ffe78c0d74\"},{\"content\":{\"connectorIds\":[\"In3\"],\"side\":\"BOTTOM\"},\"type\":\"ConnectorPlacement.EquallySpacedRectSide\",\"uuid\":\"39ef07a5-295e-41ed-8fed-e3929d4bc7fe\"}]},\"type\":\"ConnectorPlacement.EquallySpacedConnector\",\"uuid\":\"6304a2bd-355b-45e4-9c14-1a54db954efb\"}],\"packageUris\":[\"http://schema.mathworks.com/mf0/Connector/19700101\"],\"version\":\"1.0\"}"
  Phase Selector : Subsystem
      settings: PortSchema="{\"entries\":[{\"content\":{\"sides\":[{\"content\":{\"connectorIds\":[\"In1\",\"In2\",\"In3\",\"In4\",\"In5\",\"In6\",\"In7\",\"In8\"]},\"type\":\"ConnectorPlacement.EquallySpacedRectSide\",\"uuid\":\"7503323e-6ee4-44ff-b04d-f2dbeaa5c6ec\"},{\"content\":{\"connectorIds\":[\"Out1\",\"Out2\"],\"side\":\"RIGHT\"},\"type\":\"ConnectorPlacement.EquallySpacedRectSide\",\"uuid\":\"41a61174-d293-4df5-a84f-f0e93c8bdc8e\"},{\"content\":{\"connectorIds\":[],\"side\":\"TOP\"},\"type\":\"ConnectorPlacement.EquallySpacedRectSide\",\"uuid\":\"fa0b14f5-0011-4a0b-b494-1db998357d4b\"},{\"content\":{\"connectorIds\":[\"In9\"],\"side\":\"BOTTOM\"},\"type\":\"ConnectorPlacement.EquallySpacedRectSide\",\"uuid\":\"f33c2322-8ee6-4a57-a447-492661ada981\"}]},\"type\":\"ConnectorPlacement.EquallySpacedConnector\",\"uuid\":\"0b93855a-73ca-4614-8a61-5e157f0666c2\"}],\"packageUris\":[\"http://schema.mathworks.com/mf0/Connector/19700101\"],\"version\":\"1.0\"}"
  CLK1 : Outport
  CLK4 : Outport  Port=2
  CLK3 : Outport  Port=3
  CLK2 : Outport  Port=4
  wires:
  0/1 -> Phase Selector/1(0)
  225/1 -> Phase Selector/6(225)
  Phase Selector/2(CLK_s3) -> Phase Interpolator/2(CLK_s3)
  Phase Selector/1(CLK_s1) -> Phase Interpolator/1(CLK_s1)
  315/1 -> Phase Selector/8(315)
  45/1 -> Phase Selector/2(45)
  270/1 -> Phase Selector/7(270)
  135/1 -> Phase Selector/4(135)
  90/1 -> Phase Selector/3(90)
  LSB_4bit/1 -> Phase Interpolator/3(LSB_4bit)
  MSB_2bit/1 -> Phase Selector/9(MSB_2bit)
  Phase Interpolator/2(CLK3) -> CLK3/1
  Phase Interpolator/1(CLK1) -> CLK1/1
  180/1 -> Phase Selector/5(180)
  Phase Interpolator/3(CLK2) -> CLK2/1
  Phase Interpolator/4(CLK4) -> CLK4/1

== system Tx_Rx/BER_calculator/Delay Line/Subsystem32 ==
  N-1 : Inport
  Constant : Constant
  Divide : Product  Inputs=*/
  Fref : Gain  Gain=78.125e-12
  Num : Gain  Gain=8
  Relay1 : Relay
  Variable Time Delay : VariableTransportDelay  MaximumDelay=10  FixedBuffer=on
  N : Outport
  wires:
  Num/1 -> Divide/2
  N-1/1 -> Variable Time Delay/1
  Relay1/1 -> N/1
  Divide/1 -> Fref/1
  Fref/1 -> Variable Time Delay/2
  Variable Time Delay/1 -> Relay1/1
  Constant/1 -> Num/1, Divide/1

== system Tx_Rx/BER_calculator/Delay Line/Subsystem33 ==
  N-1 : Inport
  Constant : Constant
  Divide : Product  Inputs=*/
  Fref : Gain  Gain=78.125e-12
  Num : Gain  Gain=8
  Relay1 : Relay
  Variable Time Delay : VariableTransportDelay  MaximumDelay=10  FixedBuffer=on
  N : Outport
  wires:
  Num/1 -> Divide/2
  N-1/1 -> Variable Time Delay/1
  Relay1/1 -> N/1
  Divide/1 -> Fref/1
  Fref/1 -> Variable Time Delay/2
  Variable Time Delay/1 -> Relay1/1
  Constant/1 -> Num/1, Divide/1

== system Tx_Rx/BER_calculator/Delay Line/Subsystem34 ==
  N-1 : Inport
  Constant : Constant
  Divide : Product  Inputs=*/
  Fref : Gain  Gain=78.125e-12
  Num : Gain  Gain=8
  Relay1 : Relay
  Variable Time Delay : VariableTransportDelay  MaximumDelay=10  FixedBuffer=on
  N : Outport
  wires:
  Num/1 -> Divide/2
  N-1/1 -> Variable Time Delay/1
  Relay1/1 -> N/1
  Divide/1 -> Fref/1
  Fref/1 -> Variable Time Delay/2
  Variable Time Delay/1 -> Relay1/1
  Constant/1 -> Num/1, Divide/1

== system Tx_Rx/BER_calculator/Delay Line/Subsystem35 ==
  N-1 : Inport
  Constant : Constant
  Divide : Product  Inputs=*/
  Fref : Gain  Gain=78.125e-12
  Num : Gain  Gain=8
  Relay1 : Relay
  Variable Time Delay : VariableTransportDelay  MaximumDelay=10  FixedBuffer=on
  N : Outport
  wires:
  Num/1 -> Divide/2
  N-1/1 -> Variable Time Delay/1
  Relay1/1 -> N/1
  Divide/1 -> Fref/1
  Fref/1 -> Variable Time Delay/2
  Variable Time Delay/1 -> Relay1/1
  Constant/1 -> Num/1, Divide/1

== system Tx_Rx/BER_calculator/Delay Line/Subsystem36 ==
  N-1 : Inport
  Constant : Constant
  Divide : Product  Inputs=*/
  Fref : Gain  Gain=78.125e-12
  Num : Gain  Gain=8
  Relay1 : Relay
  Variable Time Delay : VariableTransportDelay  MaximumDelay=10  FixedBuffer=on
  N : Outport
  wires:
  Num/1 -> Divide/2
  N-1/1 -> Variable Time Delay/1
  Relay1/1 -> N/1
  Divide/1 -> Fref/1
  Fref/1 -> Variable Time Delay/2
  Variable Time Delay/1 -> Relay1/1
  Constant/1 -> Num/1, Divide/1

== system Tx_Rx/BER_calculator/Delay Line/Subsystem37 ==
  N-1 : Inport
  Constant : Constant
  Divide : Product  Inputs=*/
  Fref : Gain  Gain=78.125e-12
  Num : Gain  Gain=8
  Relay1 : Relay
  Variable Time Delay : VariableTransportDelay  MaximumDelay=10  FixedBuffer=on
  N : Outport
  wires:
  Num/1 -> Divide/2
  N-1/1 -> Variable Time Delay/1
  Relay1/1 -> N/1
  Divide/1 -> Fref/1
  Fref/1 -> Variable Time Delay/2
  Variable Time Delay/1 -> Relay1/1
  Constant/1 -> Num/1, Divide/1

== system Tx_Rx/BER_calculator/Delay Line/Subsystem38 ==
  N-1 : Inport
  Constant : Constant
  Divide : Product  Inputs=*/
  Fref : Gain  Gain=78.125e-12
  Num : Gain  Gain=8
  Relay1 : Relay
  Variable Time Delay : VariableTransportDelay  MaximumDelay=10  FixedBuffer=on
  N : Outport
  wires:
  Num/1 -> Divide/2
  N-1/1 -> Variable Time Delay/1
  Relay1/1 -> N/1
  Divide/1 -> Fref/1
  Fref/1 -> Variable Time Delay/2
  Variable Time Delay/1 -> Relay1/1
  Constant/1 -> Num/1, Divide/1

== system Tx_Rx/BER_calculator/Delay Line/Subsystem39 ==
  N-1 : Inport
  Constant : Constant
  Divide : Product  Inputs=*/
  Fref : Gain  Gain=78.125e-12
  Num : Gain  Gain=8
  Relay1 : Relay
  Variable Time Delay : VariableTransportDelay  MaximumDelay=10  FixedBuffer=on
  N : Outport
  wires:
  Num/1 -> Divide/2
  N-1/1 -> Variable Time Delay/1
  Relay1/1 -> N/1
  Divide/1 -> Fref/1
  Fref/1 -> Variable Time Delay/2
  Variable Time Delay/1 -> Relay1/1
  Constant/1 -> Num/1, Divide/1

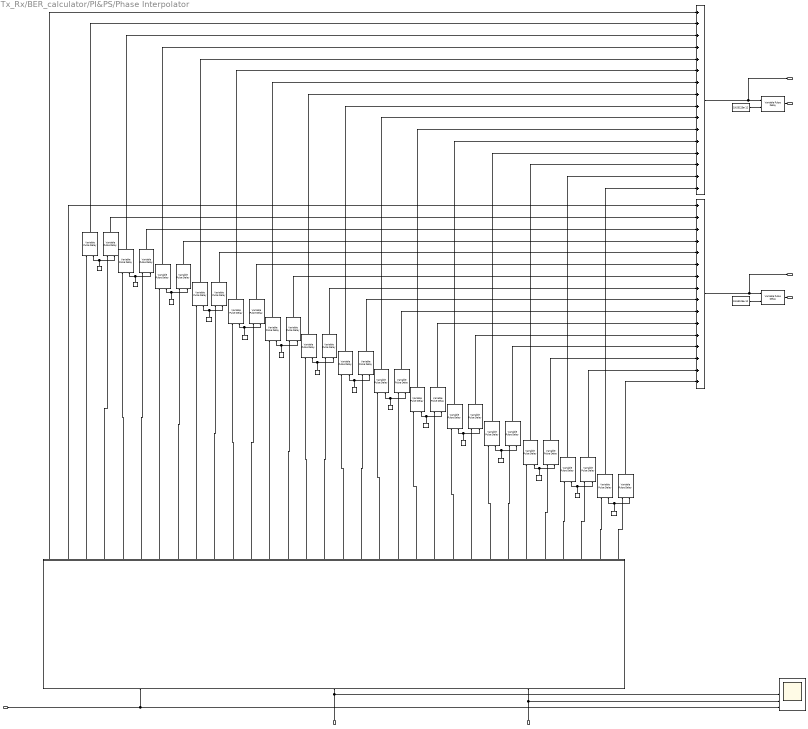
== system Tx_Rx/BER_calculator/PI&PS/Phase Interpolator ==
  CLK_s1 : Inport
  CLK_s3 : Inport  Port=2
  LSB_4bit : Inport  Port=3
  Add6 : Sum  Inputs=++++++++++++++++
  Add7 : Sum  Inputs=++++++++++++++++
  Constant26 : Constant  Value=19.53125e-12
  Constant27 : Constant  Value=0.6103515625e-12
  Constant28 : Constant  Value=2*0.6103515625e-12
  Constant29 : Constant  Value=3*0.6103515625e-12
  Constant30 : Constant  Value=4*0.6103515625e-12
  Constant31 : Constant  Value=5*0.6103515625e-12
  Constant32 : Constant  Value=6*0.6103515625e-12
  Constant33 : Constant  Value=7*0.6103515625e-12
  Constant34 : Constant  Value=8*0.6103515625e-12
  Constant35 : Constant  Value=9*0.6103515625e-12
  Constant36 : Constant  Value=10*0.6103515625e-12
  Constant37 : Constant  Value=11*0.6103515625e-12
  Constant38 : Constant  Value=12*0.6103515625e-12
  Constant39 : Constant  Value=13*0.6103515625e-12
  Constant40 : Constant  Value=14*0.6103515625e-12
  Constant41 : Constant  Value=15*0.6103515625e-12
  Constant42 : Constant  Value=19.53125e-12
  MATLAB Function : MATLAB Function  TreatAsAtomicUnit=on
  Scope : Scope  NumInputPorts=5
  Variable Pulse Delay{,1..31} (32 alike) : msbUtilities/Variable Pulse Delay  InitialInput=0  BufferSize=100
      settings: SourceProductBaseCode=AM
  CLK2 : Outport
  CLK4 : Outport  Port=2
  CLK1 : Outport  Port=3
  CLK3 : Outport  Port=4
  wires:
  Variable Pulse Delay30/1 -> Add6/16
  Constant40/1 -> Variable Pulse Delay28/2, Variable Pulse Delay29/2
  MATLAB Function/14(c6_1) -> Variable Pulse Delay13/1
  MATLAB Function/23(c11_0) -> Variable Pulse Delay22/1
  Constant34/1 -> Variable Pulse Delay17/2, Variable Pulse Delay16/2
  Constant41/1 -> Variable Pulse Delay31/2, Variable Pulse Delay30/2
  MATLAB Function/9(c4_0) -> Variable Pulse Delay8/1
  Variable Pulse Delay19/1 -> Add7/10
  Variable Pulse Delay6/1 -> Add6/4
  Constant35/1 -> Variable Pulse Delay19/2, Variable Pulse Delay18/2
  Constant27/1 -> Variable Pulse Delay2/2, Variable Pulse Delay3/2
  Variable Pulse Delay10/1 -> Add6/6
  Variable Pulse Delay25/1 -> Add7/13
  MATLAB Function/32(c15_1) -> Variable Pulse Delay31/1
  MATLAB Function/25(c12_0) -> Variable Pulse Delay24/1
  MATLAB Function/22(c10_1) -> Variable Pulse Delay21/1
  Constant33/1 -> Variable Pulse Delay15/2, Variable Pulse Delay14/2
  MATLAB Function/29(c14_0) -> Variable Pulse Delay28/1
  Constant36/1 -> Variable Pulse Delay21/2, Variable Pulse Delay20/2
  MATLAB Function/26(c12_1) -> Variable Pulse Delay25/1
  Variable Pulse Delay12/1 -> Add6/7
  Variable Pulse Delay22/1 -> Add6/12
  MATLAB Function/3(c1_0) -> Variable Pulse Delay2/1
  Constant28/1 -> Variable Pulse Delay5/2, Variable Pulse Delay4/2
  Constant31/1 -> Variable Pulse Delay11/2, Variable Pulse Delay10/2
  MATLAB Function/1(c0_0) -> Add6/1
  Constant30/1 -> Variable Pulse Delay9/2, Variable Pulse Delay8/2
  MATLAB Function/31(c15_0) -> Variable Pulse Delay30/1
  Constant38/1 -> Variable Pulse Delay25/2, Variable Pulse Delay24/2
  MATLAB Function/6(c2_1) -> Variable Pulse Delay5/1
  MATLAB Function/12(c5_1) -> Variable Pulse Delay11/1
  Variable Pulse Delay24/1 -> Add6/13
  Constant32/1 -> Variable Pulse Delay13/2, Variable Pulse Delay12/2
  MATLAB Function/17(c8_0) -> Variable Pulse Delay16/1
  MATLAB Function/15(c7_0) -> Variable Pulse Delay14/1
  Variable Pulse Delay8/1 -> Add6/5
  MATLAB Function/10(c4_1) -> Variable Pulse Delay9/1
  MATLAB Function/21(c10_0) -> Variable Pulse Delay20/1
  MATLAB Function/18(c8_1) -> Variable Pulse Delay17/1
  MATLAB Function/27(c13_0) -> Variable Pulse Delay26/1
  Variable Pulse Delay2/1 -> Add6/2
  Constant39/1 -> Variable Pulse Delay27/2, Variable Pulse Delay26/2
  MATLAB Function/2(c0_1) -> Add7/1
  Variable Pulse Delay16/1 -> Add6/9
  Variable Pulse Delay4/1 -> Add6/3
  Variable Pulse Delay18/1 -> Add6/10
  MATLAB Function/19(c9_0) -> Variable Pulse Delay18/1
  MATLAB Function/13(c6_0) -> Variable Pulse Delay12/1
  Variable Pulse Delay5/1 -> Add7/3
  Variable Pulse Delay17/1 -> Add7/9
  MATLAB Function/4(c1_1) -> Variable Pulse Delay3/1
  MATLAB Function/20(c9_1) -> Variable Pulse Delay19/1
  Variable Pulse Delay31/1 -> Add7/16
  Constant26/1 -> Variable Pulse Delay/2
  MATLAB Function/16(c7_1) -> Variable Pulse Delay15/1
  Constant42/1 -> Variable Pulse Delay1/2
  Variable Pulse Delay27/1 -> Add7/14
  Add6/1 -> CLK1/1, Variable Pulse Delay/1
  Variable Pulse Delay26/1 -> Add6/14
  Constant29/1 -> Variable Pulse Delay7/2, Variable Pulse Delay6/2
  Variable Pulse Delay13/1 -> Add7/7
  Variable Pulse Delay14/1 -> Add6/8
  Variable Pulse Delay29/1 -> Add7/15
  Variable Pulse Delay28/1 -> Add6/15
  MATLAB Function/28(c13_1) -> Variable Pulse Delay27/1
  Variable Pulse Delay3/1 -> Add7/2
  MATLAB Function/24(c11_1) -> Variable Pulse Delay23/1
  MATLAB Function/11(c5_0) -> Variable Pulse Delay10/1
  Variable Pulse Delay7/1 -> Add7/4
  MATLAB Function/5(c2_0) -> Variable Pulse Delay4/1
  Constant37/1 -> Variable Pulse Delay23/2, Variable Pulse Delay22/2
  MATLAB Function/30(c14_1) -> Variable Pulse Delay29/1
  Variable Pulse Delay21/1 -> Add7/11
  Variable Pulse Delay15/1 -> Add7/8
  Variable Pulse Delay20/1 -> Add6/11
  Variable Pulse Delay9/1 -> Add7/5
  Variable Pulse Delay11/1 -> Add7/6
  MATLAB Function/7(c3_0) -> Variable Pulse Delay6/1
  MATLAB Function/8(c3_1) -> Variable Pulse Delay7/1
  Variable Pulse Delay23/1 -> Add7/12
  Add7/1 -> CLK3/1, Variable Pulse Delay1/1
  LSB_4bit/1 -> MATLAB Function/1(LSB_4bit), Scope/5
  Variable Pulse Delay/1 -> CLK2/1
  Variable Pulse Delay1/1 -> CLK4/1
  CLK_s1/1 -> MATLAB Function/2(clk_s1), Scope/3
  CLK_s3/1 -> MATLAB Function/3(clk_s3), Scope/4

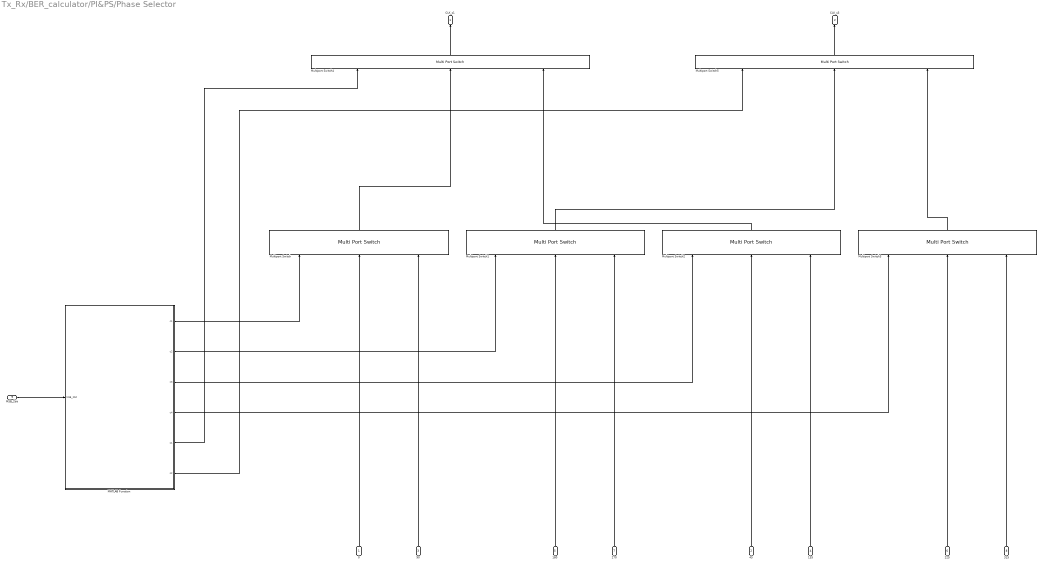
== system Tx_Rx/BER_calculator/PI&PS/Phase Selector ==
  0 : Inport
  45 : Inport  Port=2
  90 : Inport  Port=3
  135 : Inport  Port=4
  180 : Inport  Port=5
  225 : Inport  Port=6
  270 : Inport  Port=7
  315 : Inport  Port=8
  MSB_2bit : Inport  Port=9
  MATLAB Function : MATLAB Function  TreatAsAtomicUnit=on
  Multiport Switch{,1..5} (6 alike) : MultiPortSwitch  Inputs=2
  CLK_s1 : Outport
  CLK_s3 : Outport  Port=2
  wires:
  Multiport Switch1/1 -> Multiport Switch5/2
  Multiport Switch2/1 -> Multiport Switch4/3
  Multiport Switch/1 -> Multiport Switch4/2
  Multiport Switch3/1 -> Multiport Switch5/3
  225/1 -> Multiport Switch3/2
  135/1 -> Multiport Switch2/3
  0/1 -> Multiport Switch/2
  45/1 -> Multiport Switch2/2
  90/1 -> Multiport Switch/3
  315/1 -> Multiport Switch3/3
  270/1 -> Multiport Switch1/3
  180/1 -> Multiport Switch1/2
  Multiport Switch5/1 -> CLK_s3/1
  Multiport Switch4/1 -> CLK_s1/1
  MSB_2bit/1 -> MATLAB Function/1(MSB_2bit)
  MATLAB Function/1(c1) -> Multiport Switch/1
  MATLAB Function/2(c2) -> Multiport Switch1/1
  MATLAB Function/3(c3) -> Multiport Switch2/1
  MATLAB Function/4(c4) -> Multiport Switch3/1
  MATLAB Function/5(s1) -> Multiport Switch4/1
  MATLAB Function/6(s2) -> Multiport Switch5/1

== system Tx_Rx/RX/Delay Line/Subsystem32 ==
  N-1 : Inport
  Constant : Constant
  Divide : Product  Inputs=*/
  Fref : Gain  Gain=78.125e-12
  Num : Gain  Gain=8
  Relay1 : Relay
  Variable Time Delay : VariableTransportDelay  MaximumDelay=10  FixedBuffer=on
  N : Outport
  wires:
  Num/1 -> Divide/2
  N-1/1 -> Variable Time Delay/1
  Relay1/1 -> N/1
  Divide/1 -> Fref/1
  Fref/1 -> Variable Time Delay/2
  Variable Time Delay/1 -> Relay1/1
  Constant/1 -> Num/1, Divide/1

== system Tx_Rx/RX/Delay Line/Subsystem33 ==
  N-1 : Inport
  Constant : Constant
  Divide : Product  Inputs=*/
  Fref : Gain  Gain=78.125e-12
  Num : Gain  Gain=8
  Relay1 : Relay
  Variable Time Delay : VariableTransportDelay  MaximumDelay=10  FixedBuffer=on
  N : Outport
  wires:
  Num/1 -> Divide/2
  N-1/1 -> Variable Time Delay/1
  Relay1/1 -> N/1
  Divide/1 -> Fref/1
  Fref/1 -> Variable Time Delay/2
  Variable Time Delay/1 -> Relay1/1
  Constant/1 -> Num/1, Divide/1

== system Tx_Rx/RX/Delay Line/Subsystem34 ==
  N-1 : Inport
  Constant : Constant
  Divide : Product  Inputs=*/
  Fref : Gain  Gain=78.125e-12
  Num : Gain  Gain=8
  Relay1 : Relay
  Variable Time Delay : VariableTransportDelay  MaximumDelay=10  FixedBuffer=on
  N : Outport
  wires:
  Num/1 -> Divide/2
  N-1/1 -> Variable Time Delay/1
  Relay1/1 -> N/1
  Divide/1 -> Fref/1
  Fref/1 -> Variable Time Delay/2
  Variable Time Delay/1 -> Relay1/1
  Constant/1 -> Num/1, Divide/1

== system Tx_Rx/RX/Delay Line/Subsystem35 ==
  N-1 : Inport
  Constant : Constant
  Divide : Product  Inputs=*/
  Fref : Gain  Gain=78.125e-12
  Num : Gain  Gain=8
  Relay1 : Relay
  Variable Time Delay : VariableTransportDelay  MaximumDelay=10  FixedBuffer=on
  N : Outport
  wires:
  Num/1 -> Divide/2
  N-1/1 -> Variable Time Delay/1
  Relay1/1 -> N/1
  Divide/1 -> Fref/1
  Fref/1 -> Variable Time Delay/2
  Variable Time Delay/1 -> Relay1/1
  Constant/1 -> Num/1, Divide/1

== system Tx_Rx/RX/Delay Line/Subsystem36 ==
  N-1 : Inport
  Constant : Constant
  Divide : Product  Inputs=*/
  Fref : Gain  Gain=78.125e-12
  Num : Gain  Gain=8
  Relay1 : Relay
  Variable Time Delay : VariableTransportDelay  MaximumDelay=10  FixedBuffer=on
  N : Outport
  wires:
  Num/1 -> Divide/2
  N-1/1 -> Variable Time Delay/1
  Relay1/1 -> N/1
  Divide/1 -> Fref/1
  Fref/1 -> Variable Time Delay/2
  Variable Time Delay/1 -> Relay1/1
  Constant/1 -> Num/1, Divide/1

== system Tx_Rx/RX/Delay Line/Subsystem37 ==
  N-1 : Inport
  Constant : Constant
  Divide : Product  Inputs=*/
  Fref : Gain  Gain=78.125e-12
  Num : Gain  Gain=8
  Relay1 : Relay
  Variable Time Delay : VariableTransportDelay  MaximumDelay=10  FixedBuffer=on
  N : Outport
  wires:
  Num/1 -> Divide/2
  N-1/1 -> Variable Time Delay/1
  Relay1/1 -> N/1
  Divide/1 -> Fref/1
  Fref/1 -> Variable Time Delay/2
  Variable Time Delay/1 -> Relay1/1
  Constant/1 -> Num/1, Divide/1

== system Tx_Rx/RX/Delay Line/Subsystem38 ==
  N-1 : Inport
  Constant : Constant  SampleTime=-1
  Divide : Product  Inputs=*/
  Fref : Gain  Gain=78.125e-12
  Num : Gain  Gain=8
  Relay1 : Relay
  Variable Time Delay : VariableTransportDelay  MaximumDelay=10  FixedBuffer=on
  N : Outport
  wires:
  N-1/1 -> Variable Time Delay/1
  Relay1/1 -> N/1
  Variable Time Delay/1 -> Relay1/1
  Fref/1 -> Variable Time Delay/2
  Divide/1 -> Fref/1
  Num/1 -> Divide/2
  Constant/1 -> Num/1, Divide/1

== system Tx_Rx/RX/Delay Line/Subsystem39 ==
  N-1 : Inport
  Constant : Constant
  Divide : Product  Inputs=*/
  Fref : Gain  Gain=78.125e-12
  Num : Gain  Gain=8
  Relay1 : Relay
  Variable Time Delay : VariableTransportDelay  MaximumDelay=10  FixedBuffer=on
  N : Outport
  wires:
  Num/1 -> Divide/2
  N-1/1 -> Variable Time Delay/1
  Relay1/1 -> N/1
  Divide/1 -> Fref/1
  Fref/1 -> Variable Time Delay/2
  Variable Time Delay/1 -> Relay1/1
  Constant/1 -> Num/1, Divide/1
